simulink model "SimulinkMonteCarlo"  (R2013b)
settings: Solver=FixedStepDiscrete  StartTime=0.0  StopTime=20  FixedStep=0.01  RelTol=1e-3
undefined symbols (not defined in the file or in its folder): Ad, Bd, C
settings Model: Creator=ThiagoCordeiro  LastModifiedBy=ThiagoFelippe

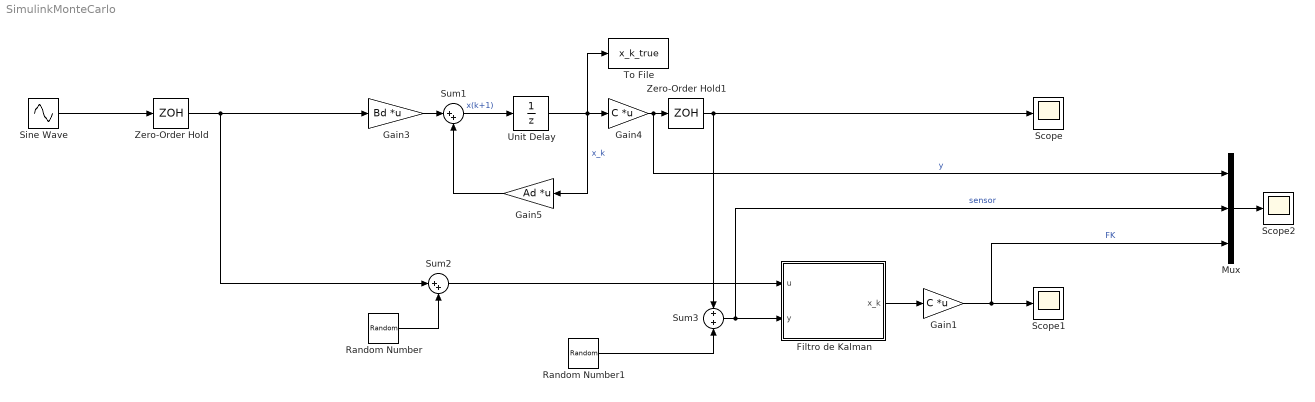
== system SimulinkMonteCarlo ==
  Filtro de Kalman : Subsystem
  Gain1 : Gain  Gain=C  Multiplication=Matrix(K*u)
  Gain3 : Gain  Gain=Bd  Multiplication=Matrix(K*u)
  Gain4 : Gain  Gain=C  Multiplication=Matrix(K*u)
  Gain5 : Gain  Gain=Ad  Multiplication=Matrix(K*u)
  Mux : Mux  Inputs=3
  Random Number : RandomNumber  Seed=round(rand(1)*(2^32-1))  SampleTime=0.01
  Random Number1 : RandomNumber  Seed=round(rand(1)*(2^32-1))  SampleTime=0.01
  Scope : Scope
  Scope1 : Scope
  Scope2 : Scope
      settings: ShowLegends=on  SaveName=ScopeData2
  Sine Wave : Sin  Phase=pi/2  SampleTime=0
  Sum1 : Sum  Inputs=|++
  Sum2 : Sum  Inputs=|++
  Sum3 : Sum  Inputs=+|+
  To File : ToFile  Filename=x_k_true  MatrixName=x_k_true  SaveFormat=Timeseries
  Unit Delay : UnitDelay  InitialCondition=[0;0]  SampleTime=-1
  Zero-Order Hold : ZeroOrderHold  SampleTime=0.01
  Zero-Order Hold1 : ZeroOrderHold  SampleTime=0.01
  wires:
  Gain3/1 -> Sum1/1
  Sum1/1 -> Unit Delay/1  "x(k+1)"
  Unit Delay/1 -> To File/1, Gain4/1, Gain5/1  "x_k"
  Gain5/1 -> Sum1/2
  Filtro de Kalman/1(x_k) -> Gain1/1
  Gain1/1 -> Mux/3, Scope1/1  "FK"
  Mux/1 -> Scope2/1
  Zero-Order Hold/1 -> Sum2/1, Gain3/1
  Sum2/1 -> Filtro de Kalman/1(u)
  Random Number/1 -> Sum2/2
  Sum3/1 -> Mux/2, Filtro de Kalman/2(y)  "sensor"
  Random Number1/1 -> Sum3/2
  Zero-Order Hold1/1 -> Scope/1, Sum3/1
  Gain4/1 -> Mux/1, Zero-Order Hold1/1  "y"
  Sine Wave/1 -> Zero-Order Hold/1

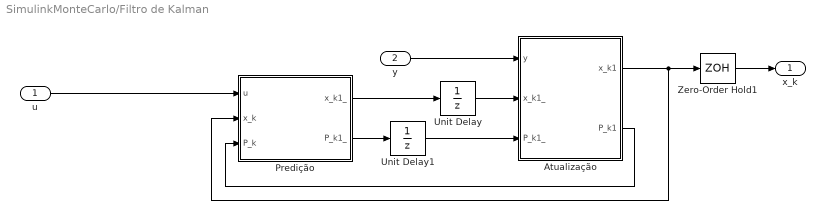
== system SimulinkMonteCarlo/Filtro de Kalman ==
  u : Inport
  y : Inport  Port=2
  Atualização : Subsystem
  Predição : Subsystem
  Unit Delay : UnitDelay  InitialCondition=4*randn(2,1)  SampleTime=0.01
  Unit Delay1 : UnitDelay  InitialCondition=[16 0; 0 16]  SampleTime=0.01
  Zero-Order Hold1 : ZeroOrderHold  SampleTime=0.01
  x_k : Outport
  wires:
  u/1 -> Predição/1(u)
  y/1 -> Atualização/1(y)
  Atualização/1(x_k1) -> Predição/2(x_k), Zero-Order Hold1/1
  Atualização/2(P_k1) -> Predição/3(P_k)
  Zero-Order Hold1/1 -> x_k/1
  Predição/2(P_k1_) -> Unit Delay1/1
  Unit Delay1/1 -> Atualização/3(P_k1_)
  Unit Delay/1 -> Atualização/2(x_k1_)
  Predição/1(x_k1_) -> Unit Delay/1

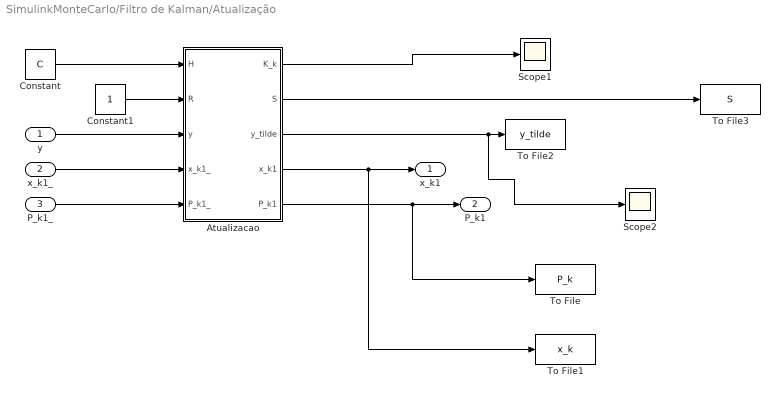
== system SimulinkMonteCarlo/Filtro de Kalman/Atualização ==
  y : Inport
  x_k1_ : Inport  Port=2
  P_k1_ : Inport  Port=3
  Atualizacao : MATLAB Function  TreatAsAtomicUnit=on  SystemSampleTime=0.01
  Constant : Constant  Value=C  VectorParams1D=off
  Constant1 : Constant
  Scope1 : Scope
      settings: SaveName=ScopeData3
  Scope2 : Scope
      settings: SaveName=ScopeData5
  To File : ToFile  Filename=P_k  MatrixName=P_k  SaveFormat=Timeseries
  To File1 : ToFile  Filename=x_k  MatrixName=x_k  SaveFormat=Timeseries
  To File2 : ToFile  Filename=y_tilde  MatrixName=y_tilde  SaveFormat=Timeseries
  To File3 : ToFile  Filename=S  MatrixName=S  SaveFormat=Timeseries
  x_k1 : Outport
  P_k1 : Outport  Port=2
  wires:
  y/1 -> Atualizacao/3(y)
  x_k1_/1 -> Atualizacao/4(x_k1_)
  P_k1_/1 -> Atualizacao/5(P_k1_)
  Atualizacao/4(x_k1) -> To File1/1, x_k1/1
  Atualizacao/5(P_k1) -> To File/1, P_k1/1
  Constant/1 -> Atualizacao/1(H)
  Constant1/1 -> Atualizacao/2(R)
  Atualizacao/1(K_k) -> Scope1/1
  Atualizacao/2(S) -> To File3/1
  Atualizacao/3(y_tilde) -> To File2/1, Scope2/1

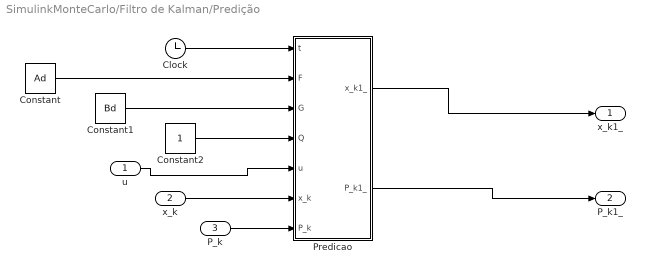
== system SimulinkMonteCarlo/Filtro de Kalman/Predição ==
  u : Inport
  x_k : Inport  Port=2
  P_k : Inport  Port=3
  Clock : Clock
  Constant : Constant  Value=Ad
  Constant1 : Constant  Value=Bd  VectorParams1D=off
  Constant2 : Constant
  Predicao : MATLAB Function  TreatAsAtomicUnit=on  SystemSampleTime=0.01
  x_k1_ : Outport
  P_k1_ : Outport  Port=2
  wires:
  u/1 -> Predicao/5(u)
  x_k/1 -> Predicao/6(x_k)
  P_k/1 -> Predicao/7(P_k)
  Constant/1 -> Predicao/2(F)
  Constant1/1 -> Predicao/3(G)
  Constant2/1 -> Predicao/4(Q)
  Predicao/1(x_k1_) -> x_k1_/1
  Predicao/2(P_k1_) -> P_k1_/1
  Clock/1 -> Predicao/1(t)

== matlab function SimulinkMonteCarlo/Filtro de Kalman/Atualização/Atualizacao ==
  data: H input; R input; K_k output; S output; y_tilde output; y input; x_k1_ input; P_k1_ input; x_k1 output; P_k1 output
function [K_k, S, y_tilde, x_k1, P_k1] = fcn(H, R, y, x_k1_, P_k1_)
%#codegen

% Trecho abaixo nao depende nem do estado estimado, nem da medida obtida,
% entao pode ser calculado offline e armazenado em tabela
S = H * P_k1_ * H' + R;
Pxy = P_k1_ * H';
K_k  =  Pxy / S;
KH = K_k*H;
I = eye(size(KH));
I_KH = I - KH;
P_k1 = I_KH * P_k1_ * I_KH' + K_k * R * K_k';
% --- fim do trecho que pode ser calculado offline

y_hat = H * x_k1_;
y_tilde = y - y_hat;
x_k1 = x_k1_ + K_k * y_tilde;

== matlab function SimulinkMonteCarlo/Filtro de Kalman/Predição/Predicao ==
  data: t input; F input; G input; Q input; u input; x_k1_ output; x_k input; P_k input; P_k1_ output
function [x_k1_,P_k1_] = fcn(t, F, G, Q, u, x_k, P_k)
%#codegen
if t >= 0
    x_k1_ = F*x_k + G*u;
    P_k1_ = F*P_k*F' + G*Q*G';
else
    x_k1_ = x_k;
    P_k1_ = P_k;
end
